simulink model "Active_suspension_system_of_a_quarter_car"  (R2019a)
settings: Solver=VariableStepAuto  StartTime=0.0  StopTime=20  RelTol=1e-3
libraries: simulink x1
settings Model: Creator=Arun  LastModifiedBy=Arun

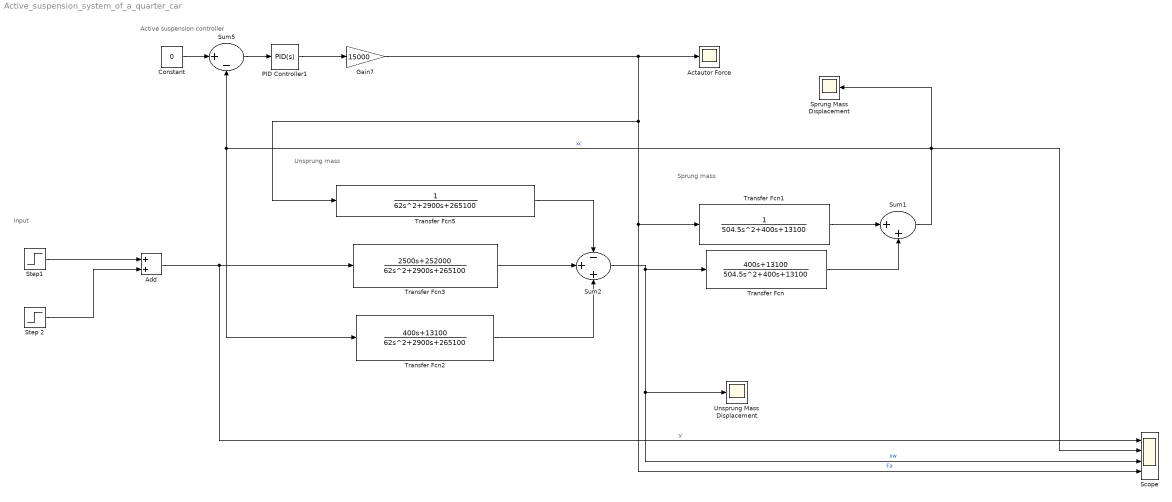
== system Active_suspension_system_of_a_quarter_car ==
  note: Active suspension controller
  note: Sprung mass
  note: Unsprung mass
  note: Input
  Actautor Force : Scope
  Add : Sum
  Constant : Constant  Value=0
  Gain7 : Gain  Gain=15000
  PID Controller1 : simulink/Continuous/PID Controller  Controller=PID  Form=Parallel  TimeDomain=Continuous-time  SampleTime=-1  IntegratorMethod=Forward Euler  FilterMethod=Forward Euler  ControllerParametersSource=internal  P=4.9751  I=4.9489  D=0.3614  UseFilter=on  N=414.1968  TunerSelectOption=Transfer Function Based (PID Tuner App)  InitialConditionSource=internal  InitialConditionForIntegrator=0  InitialConditionForFilter=0  DifferentiatorICPrevScaledInput=0  ExternalReset=none  TrackingMode=off  Kt=1  LimitOutput=off  UpperSaturationLimit=inf  LowerSaturationLimit=-inf  LinearizeAsGain=on  AntiWindupMode=none  Kb=1  POutMin=[]  POutMax=[]  IOutMin=[]  IOutMax=[]  DOutMin=[]  DOutMax=[]  NOutMin=[]  NOutMax=[]  SumOutMin=[]  SumOutMax=[]  SaturationOutMin=[]  SaturationOutMax=[]  PParamMin=[]  PParamMax=[]  IParamMin=[]  IParamMax=[]  DParamMin=[]  DParamMax=[]  NParamMin=[]  NParamMax=[]  KbParamMin=[]  KbParamMax=[]  KtParamMin=[]  KtParamMax=[]  KbOutMin=[]  KbOutMax=[]  KtOutMin=[]  KtOutMax=[]  IntegratorOutMin=[]  IntegratorOutMax=[]  FilterOutMin=[]  FilterOutMax=[]  SumI1OutMin=[]  SumI1OutMax=[]  SumI2OutMin=[]  SumI2OutMax=[]  SumI3OutMin=[]  SumI3OutMax=[]  SumI4OutMin=[]  SumI4OutMax=[]  SumDOutMin=[]  SumDOutMax=[]  DifferentiatorOutMin=[]  DifferentiatorOutMax=[]  FilterDiffOutCoefMin=[]  FilterDiffOutCoefMax=[]  ReciprocalOutMin=[]  ReciprocalOutMax=[]  SumDenOutMin=[]  SumDenOutMax=[]  SumNumOutMin=[]  SumNumOutMax=[]  DivideOutMin=[]  DivideOutMax=[]  IntegratorContinuousStateAttributes=''  IntegratorStateMustResolveToSignalObject=off  IntegratorRTWStateStorageClass=Auto  FilterContinuousStateAttributes=''  FilterStateMustResolveToSignalObject=off  FilterRTWStateStorageClass=Auto  ParallelPVariant=InternalParameters  IdealPVariant=Disabled  IVariant=InternalParameters  DVariant=InternalParameters  IntegratorVariant=Continuous  SatVariant=Disabled  AWVariant=Passthrough  PCopyVariant=Disabled  TRVariant=Disabled  FdbkBlocksVariant=Forward  IdealPFdbkVariant=Disabled  SatFdbkVariant=Disabled  DerivativeFilterVariant=ContFilter  NVariant=InternalParameters  NCopyVariant=Disabled  FilterICVariant=InternalICsFilter  IntegratorICVariant=InternalICs  ExternalResetVariant=Disabled  TRSumVariant=Passthrough  SumFdbkVariant=Disabled  SumVariant=Sum_PID
  Scope : Scope  NumInputPorts=4
  Sprung Mass Displacement : Scope
  Step 2 : Step  Time=5  After=-10  SampleTime=0
  Step1 : Step  Time=3  After=10  SampleTime=0
  Sum1 : Sum  Inputs=|++
  Sum2 : Sum  Inputs=-++
  Sum5 : Sum  Inputs=|+-
  Transfer Fcn : TransferFcn  Numerator="[400  13100]"  Denominator="[504.5  400  13100]"
  Transfer Fcn1 : TransferFcn  Denominator="[504.5  400  13100]"
  Transfer Fcn2 : TransferFcn  Numerator=[400 13100]  Denominator="[62  2900  265100]"
  Transfer Fcn3 : TransferFcn  Numerator=[2500 252000]  Denominator="[62  2900  265100]"
  Transfer Fcn5 : TransferFcn  Denominator="[62  2900  265100]"
  Unsprung Mass Displacement : Scope
  wires:
  PID Controller1/1 -> Gain7/1
  Transfer Fcn1/1 -> Sum1/1
  Transfer Fcn/1 -> Sum1/2
  Gain7/1 -> Actautor Force/1, Scope/4, Transfer Fcn1/1, Transfer Fcn5/1  "Fa"
  Sum2/1 -> Transfer Fcn/1, Scope/3, Unsprung Mass Displacement/1  "xw"
  Sum1/1 -> Scope/2, Sprung Mass Displacement/1, Sum5/2, Transfer Fcn2/1  "xc"
  Add/1 -> Scope/1, Transfer Fcn3/1  "y"
  Transfer Fcn2/1 -> Sum2/3
  Transfer Fcn3/1 -> Sum2/2
  Transfer Fcn5/1 -> Sum2/1
  Sum5/1 -> PID Controller1/1
  Constant/1 -> Sum5/1
  Step1/1 -> Add/1
  Step 2/1 -> Add/2
